simulink model "segnonlinear"  (R2020a)
settings: Solver=VariableStepAuto  StartTime=0.0  StopTime=t_stop  RelTol=1e-3
values from neighbouring files (symbols this model uses):
  K_lqr = lqr(A,B,Q,R)    [segway_m.m]
  X0 = [0; 0; 2*pi/180; 0]    [segway_m.m]
settings Model: Creator=super  LastModifiedBy=super
settings DataIOCC: SaveFormat=Array  SaveOutput=off  SignalLogging=off  DSMLogging=off  SaveTime=off  ReturnWorkspaceOutputs=off

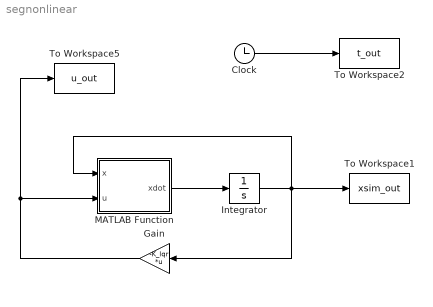
== system segnonlinear ==
  Clock : Clock
  Gain : Gain  Gain=-K_lqr  Multiplication=Matrix(K*u)
  Integrator : Integrator  InitialCondition=X0
  MATLAB Function : MATLAB Function  TreatAsAtomicUnit=on
  To Workspace1 : ToWorkspace  VariableName=xsim_out  SampleTime=-1
      settings: Save2DSignal=2-D array (concatenate along first dimension)
  To Workspace2 : ToWorkspace  VariableName=t_out  SampleTime=-1
      settings: Save2DSignal=2-D array (concatenate along first dimension)
  To Workspace5 : ToWorkspace  VariableName=u_out  SampleTime=-1
      settings: Save2DSignal=2-D array (concatenate along first dimension)
  wires:
  Clock/1 -> To Workspace2/1
  Integrator/1 -> MATLAB Function/1(x), To Workspace1/1, Gain/1
  MATLAB Function/1(xdot) -> Integrator/1
  Gain/1 -> MATLAB Function/2(u), To Workspace5/1

== matlab function segnonlinear/MATLAB Function ==
  data: x input size=[4 1]; xdot output; u input size=[1 1]
function xdot=segode2(x, u)

xdot=segode2([],x, u);
